simulink model "spacecraft"  (R2022b)
settings: Solver=FixedStepAuto  StartTime=0.0  StopTime=t_max  FixedStep=timestep  RelTol=1e-3
values from neighbouring files (symbols this model uses):
  J = Jx    (= 1150)    [script.m]
  Ka = 2    [script.m]
  step_v = 1    [script.m]
  Ta = 0.5    [script.m]
  timestep = t_max/1e6    (= 0.001)    [script.m]
libraries: simulink x1
settings Model: Creator=mluser  LastModifiedBy=mluser

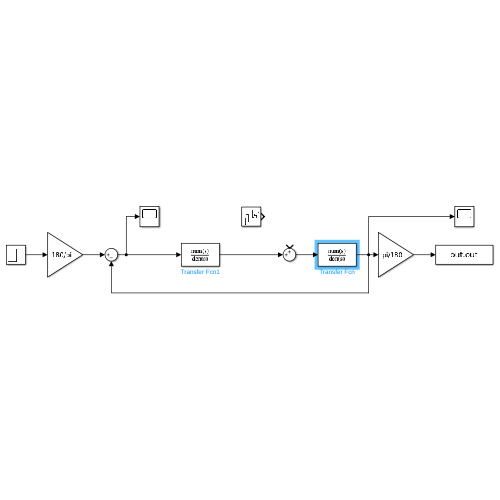
[thumbnail: Simulink's stored preview of the top-level diagram]
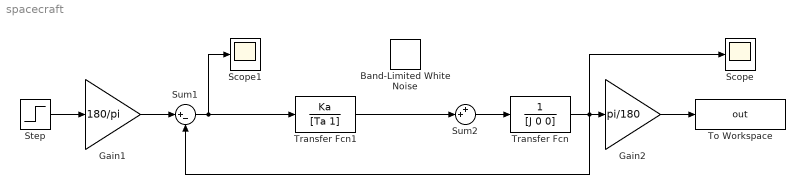
== system spacecraft ==
  Band-Limited White Noise : simulink/Sources/Band-Limited White Noise  Cov=[0.1]  Ts=timestep  seed=[23341]
  Gain1 : Gain  Gain=180/pi
  Gain2 : Gain  Gain=pi/180
  Scope : Scope
  Scope1 : Scope
  Step : Step  Time=step_v  SampleTime=0
  Sum1 : Sum  Inputs=|+-
  Sum2 : Sum  Inputs=++|
  To Workspace : ToWorkspace  VariableName=out  SampleTime=-1
  Transfer Fcn : TransferFcn  Denominator=[J 0 0]
  Transfer Fcn1 : TransferFcn  Numerator=Ka  Denominator=[Ta 1]
  wires:
  Step/1 -> Gain1/1
  Sum2/1 -> Transfer Fcn/1
  Sum1/1 -> Transfer Fcn1/1, Scope1/1
  Gain1/1 -> Sum1/1
  Transfer Fcn/1 -> Gain2/1, Sum1/2, Scope/1
  Transfer Fcn1/1 -> Sum2/2
  Gain2/1 -> To Workspace/1
